simulink model "ocxo_temp_ctrl"  (R2024b)
settings: Solver=VariableStepAuto  StartTime=0.0  StopTime=10.0  RelTol=1e-3
libraries: simulink x1, fuzblock x1
settings Model: Creator=Danfi  LastModifiedBy=Danfi

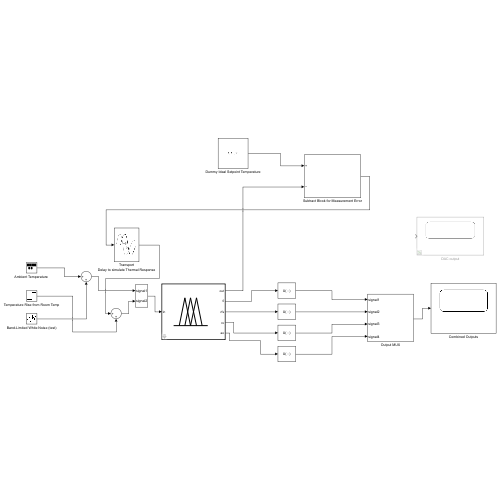
[thumbnail: Simulink's stored preview of the top-level diagram]
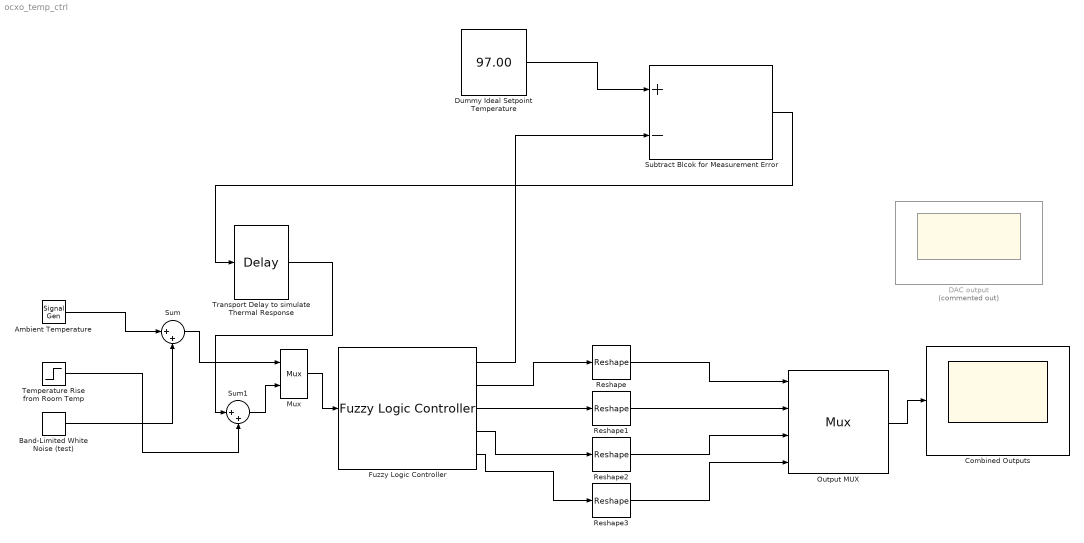
== system ocxo_temp_ctrl ==
  "Ambient Temperature " : SignalGenerator  Amplitude=3.5  Frequency=0.001
  Band-Limited White Noise (test) : simulink/Sources/Band-Limited White Noise  Cov=[0.01]  Ts=0.1  seed=[23341]
  Combined Outputs : Scope
  DAC output : Scope  Commented=on
  Dummy Ideal Setpoint Temperature : Constant  Value=97.00
  Fuzzy Logic Controller : fuzblock/Fuzzy Logic  Controller  FIS='OCXO_Type2_Sugeno_1.fis'  OutputSampleNumber=101  DataType=double  FuzzifiedInputs=on  RuleFiringStrengths=on  RuleOutputs=on  AggregatedOutputs=on  SimulateUsing=Interpreted execution  OutOfRangeInputValueMessage=warning  NoRuleFiredMessage=warning  EmptyOutputFuzzySetMessage=warning
  Mux : Mux  Inputs=2
      settings: DisplayOption=signals
  Output MUX : Mux
      settings: DisplayOption=signals
  Reshape{,1..3} (4 alike) : Reshape
  Subtract Blcok for Measurement Error : Sum  Inputs=+-  OutDataTypeStr=double  AccumDataTypeStr=double
  Sum : Sum  Inputs=|++
  Sum1 : Sum  Inputs=|++
  Temperature Rise from Room Temp : Step  Time=0  Before=25  After=97  SampleTime=120
  Transport Delay to simulate Thermal Response : TransportDelay  DelayTime=10  InitialOutput=25
  wires:
  Output MUX/1 -> Combined Outputs/1
  Fuzzy Logic Controller/1 -> Subtract Blcok for Measurement Error/2
  Dummy Ideal Setpoint Temperature/1 -> Subtract Blcok for Measurement Error/1
  Subtract Blcok for Measurement Error/1 -> Transport Delay to simulate Thermal Response/1
  Fuzzy Logic Controller/2 -> Reshape/1
  Reshape/1 -> Output MUX/1
  Fuzzy Logic Controller/3 -> Reshape1/1
  Reshape1/1 -> Output MUX/2
  Fuzzy Logic Controller/4 -> Reshape2/1
  Reshape2/1 -> Output MUX/3
  Fuzzy Logic Controller/5 -> Reshape3/1
  Reshape3/1 -> Output MUX/4
  "Ambient Temperature "/1 -> Sum/1
  Band-Limited White Noise (test)/1 -> Sum/2
  Temperature Rise from Room Temp/1 -> Sum1/2
  Transport Delay to simulate Thermal Response/1 -> Sum1/1
  Sum/1 -> Mux/1
  Sum1/1 -> Mux/2
  Mux/1 -> Fuzzy Logic Controller/1
